simulink model "Ex2"  (R2013a)
settings: Solver=ode45  StartTime=0.0  StopTime=10.0  RelTol=1e-3
settings Model: Creator=Sudip Sinha  LastModifiedBy=Sudip Sinha

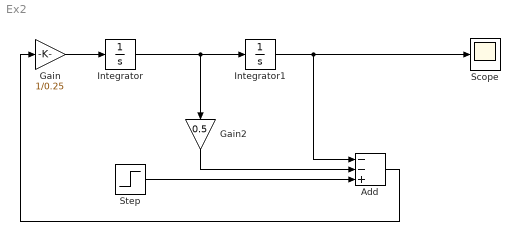
== system Ex2 ==
  Add : Sum  Inputs=--+
  Gain : Gain  Gain=1/0.25
  Gain2 : Gain  Gain=0.5
  Integrator : Integrator
  Integrator1 : Integrator
  Scope : Scope
  Step : Step  After=3  SampleTime=0
  wires:
  Integrator/1 -> Gain2/1, Integrator1/1
  Gain/1 -> Integrator/1
  Gain2/1 -> Add/2
  Integrator1/1 -> Add/1, Scope/1
  Step/1 -> Add/3
  Add/1 -> Gain/1
